simulink model "gm_uz_SVPWM_6ph"  (R2024a)
settings: Solver=FixedStepDiscrete  StartTime=0.0  StopTime=0.0004  RelTol=1e-3
undefined symbols (not defined in the file or in its folder): f_FPGA_clk, T_FPGA_clk
libraries: hdlsllib x7, simulink x1
(part 2 of 2)

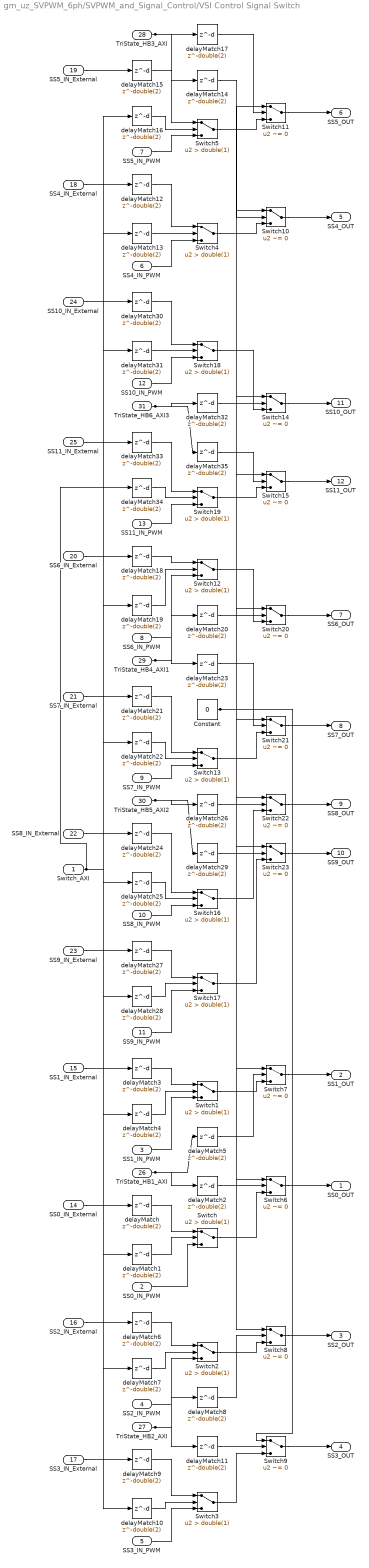
== system gm_uz_SVPWM_6ph/SVPWM_and_Signal_Control/VSI Control Signal Switch ==
  Switch_AXI : Inport  OutDataTypeStr=fixdt(0, 2, 0)  PortDimensions=1  SampleTime=1e-08
  SS0_IN_PWM : Inport  Port=2  OutDataTypeStr=fixdt(0, 1, 0)  PortDimensions=1  SampleTime=1e-08
  SS1_IN_PWM : Inport  Port=3  OutDataTypeStr=fixdt(0, 1, 0)  PortDimensions=1  SampleTime=1e-08
  SS2_IN_PWM : Inport  Port=4  OutDataTypeStr=fixdt(0, 1, 0)  PortDimensions=1  SampleTime=1e-08
  SS3_IN_PWM : Inport  Port=5  OutDataTypeStr=fixdt(0, 1, 0)  PortDimensions=1  SampleTime=1e-08
  SS4_IN_PWM : Inport  Port=6  OutDataTypeStr=fixdt(0, 1, 0)  PortDimensions=1  SampleTime=1e-08
  SS5_IN_PWM : Inport  Port=7  OutDataTypeStr=fixdt(0, 1, 0)  PortDimensions=1  SampleTime=1e-08
  SS6_IN_PWM : Inport  Port=8  OutDataTypeStr=fixdt(0, 1, 0)  PortDimensions=1  SampleTime=1e-08
  SS7_IN_PWM : Inport  Port=9  OutDataTypeStr=fixdt(0, 1, 0)  PortDimensions=1  SampleTime=1e-08
  SS8_IN_PWM : Inport  Port=10  OutDataTypeStr=fixdt(0, 1, 0)  PortDimensions=1  SampleTime=1e-08
  SS9_IN_PWM : Inport  Port=11  OutDataTypeStr=fixdt(0, 1, 0)  PortDimensions=1  SampleTime=1e-08
  SS10_IN_PWM : Inport  Port=12  OutDataTypeStr=fixdt(0, 1, 0)  PortDimensions=1  SampleTime=1e-08
  SS11_IN_PWM : Inport  Port=13  OutDataTypeStr=fixdt(0, 1, 0)  PortDimensions=1  SampleTime=1e-08
  SS0_IN_External : Inport  Port=14  OutDataTypeStr=boolean  PortDimensions=1  SampleTime=1e-08
  SS1_IN_External : Inport  Port=15  OutDataTypeStr=boolean  PortDimensions=1  SampleTime=1e-08
  SS2_IN_External : Inport  Port=16  OutDataTypeStr=boolean  PortDimensions=1  SampleTime=1e-08
  SS3_IN_External : Inport  Port=17  OutDataTypeStr=boolean  PortDimensions=1  SampleTime=1e-08
  SS4_IN_External : Inport  Port=18  OutDataTypeStr=boolean  PortDimensions=1  SampleTime=1e-08
  SS5_IN_External : Inport  Port=19  OutDataTypeStr=boolean  PortDimensions=1  SampleTime=1e-08
  SS6_IN_External : Inport  Port=20  OutDataTypeStr=boolean  PortDimensions=1  SampleTime=1e-08
  SS7_IN_External : Inport  Port=21  OutDataTypeStr=boolean  PortDimensions=1  SampleTime=1e-08
  SS8_IN_External : Inport  Port=22  OutDataTypeStr=boolean  PortDimensions=1  SampleTime=1e-08
  SS9_IN_External : Inport  Port=23  OutDataTypeStr=boolean  PortDimensions=1  SampleTime=1e-08
  SS10_IN_External : Inport  Port=24  OutDataTypeStr=boolean  PortDimensions=1  SampleTime=1e-08
  SS11_IN_External : Inport  Port=25  OutDataTypeStr=boolean  PortDimensions=1  SampleTime=1e-08
  TriState_HB1_AXI : Inport  Port=26  OutDataTypeStr=boolean  PortDimensions=1  SampleTime=1e-08
  TriState_HB2_AXI : Inport  Port=27  OutDataTypeStr=boolean  PortDimensions=1  SampleTime=1e-08
  TriState_HB3_AXI : Inport  Port=28  OutDataTypeStr=boolean  PortDimensions=1  SampleTime=1e-08
  TriState_HB4_AXI1 : Inport  Port=29  OutDataTypeStr=boolean  PortDimensions=1  SampleTime=1e-08
  TriState_HB5_AXI2 : Inport  Port=30  OutDataTypeStr=boolean  PortDimensions=1  SampleTime=1e-08
  TriState_HB6_AXI3 : Inport  Port=31  OutDataTypeStr=boolean  PortDimensions=1  SampleTime=1e-08
  Constant : Constant  Value=0  OutDataTypeStr=boolean  SampleTime=1e-08
  Switch{,1..5,12..13,16..19} (12 alike) : Switch  Criteria=u2 > Threshold  Threshold=double(1)  OutDataTypeStr=boolean  SampleTime=1e-08  SaturateOnIntegerOverflow=off  InputSameDT=off
  Switch{6..11,14..15,20..23} (12 alike) : Switch  Criteria=u2 ~= 0  Threshold=double(0)  OutDataTypeStr=boolean  SampleTime=1e-08  SaturateOnIntegerOverflow=off  InputSameDT=off
  delayMatch{,1..35} (36 alike) : Delay  DelayLength=double(2)  InitialCondition=0  SampleTime=1e-08
  SS0_OUT : Outport  SampleTime=1e-08  VectorParamsAs1DForOutWhenUnconnected=off
  SS1_OUT : Outport  Port=2  SampleTime=1e-08  VectorParamsAs1DForOutWhenUnconnected=off
  SS2_OUT : Outport  Port=3  SampleTime=1e-08  VectorParamsAs1DForOutWhenUnconnected=off
  SS3_OUT : Outport  Port=4  SampleTime=1e-08  VectorParamsAs1DForOutWhenUnconnected=off
  SS4_OUT : Outport  Port=5  SampleTime=1e-08  VectorParamsAs1DForOutWhenUnconnected=off
  SS5_OUT : Outport  Port=6  SampleTime=1e-08  VectorParamsAs1DForOutWhenUnconnected=off
  SS6_OUT : Outport  Port=7  SampleTime=1e-08  VectorParamsAs1DForOutWhenUnconnected=off
  SS7_OUT : Outport  Port=8  SampleTime=1e-08  VectorParamsAs1DForOutWhenUnconnected=off
  SS8_OUT : Outport  Port=9  SampleTime=1e-08  VectorParamsAs1DForOutWhenUnconnected=off
  SS9_OUT : Outport  Port=10  SampleTime=1e-08  VectorParamsAs1DForOutWhenUnconnected=off
  SS10_OUT : Outport  Port=11  SampleTime=1e-08  VectorParamsAs1DForOutWhenUnconnected=off
  SS11_OUT : Outport  Port=12  SampleTime=1e-08  VectorParamsAs1DForOutWhenUnconnected=off
  wires:
  delayMatch1/1 -> Switch/2
  SS0_IN_PWM/1 -> Switch/3
  SS1_IN_PWM/1 -> Switch1/3
  SS2_IN_PWM/1 -> Switch2/3
  SS3_IN_PWM/1 -> Switch3/3
  SS4_IN_PWM/1 -> Switch4/3
  SS5_IN_PWM/1 -> Switch5/3
  SS6_IN_PWM/1 -> Switch12/3
  SS7_IN_PWM/1 -> Switch13/3
  SS8_IN_PWM/1 -> Switch16/3
  SS9_IN_PWM/1 -> Switch17/3
  SS10_IN_PWM/1 -> Switch18/3
  SS11_IN_PWM/1 -> Switch19/3
  delayMatch/1 -> Switch/1
  delayMatch3/1 -> Switch1/1
  delayMatch6/1 -> Switch2/1
  delayMatch9/1 -> Switch3/1
  delayMatch12/1 -> Switch4/1
  delayMatch15/1 -> Switch5/1
  delayMatch18/1 -> Switch12/1
  delayMatch21/1 -> Switch13/1
  delayMatch24/1 -> Switch16/1
  delayMatch27/1 -> Switch17/1
  delayMatch30/1 -> Switch18/1
  delayMatch33/1 -> Switch19/1
  delayMatch2/1 -> Switch6/2
  delayMatch8/1 -> Switch8/2
  delayMatch14/1 -> Switch10/2
  delayMatch20/1 -> Switch20/2
  delayMatch26/1 -> Switch22/2
  delayMatch32/1 -> Switch14/2
  Constant/1 -> Switch9/1, Switch8/1, Switch7/1, Switch6/1, Switch23/1, Switch22/1, Switch21/1, Switch20/1, Switch15/1, Switch14/1, Switch11/1, Switch10/1
  Switch/1 -> Switch6/3
  Switch1/1 -> Switch7/3
  Switch10/1 -> SS4_OUT/1
  Switch11/1 -> SS5_OUT/1
  Switch12/1 -> Switch20/3
  Switch13/1 -> Switch21/3
  Switch14/1 -> SS10_OUT/1
  Switch15/1 -> SS11_OUT/1
  Switch16/1 -> Switch22/3
  Switch17/1 -> Switch23/3
  Switch18/1 -> Switch14/3
  Switch19/1 -> Switch15/3
  Switch2/1 -> Switch8/3
  Switch20/1 -> SS6_OUT/1
  Switch21/1 -> SS7_OUT/1
  Switch22/1 -> SS8_OUT/1
  Switch23/1 -> SS9_OUT/1
  Switch3/1 -> Switch9/3
  Switch4/1 -> Switch10/3
  Switch5/1 -> Switch11/3
  Switch6/1 -> SS0_OUT/1
  Switch7/1 -> SS1_OUT/1
  Switch8/1 -> SS2_OUT/1
  Switch9/1 -> SS3_OUT/1
  SS0_IN_External/1 -> delayMatch/1
  delayMatch4/1 -> Switch1/2
  delayMatch5/1 -> Switch7/2
  SS1_IN_External/1 -> delayMatch3/1
  delayMatch7/1 -> Switch2/2
  TriState_HB1_AXI/1 -> delayMatch5/1, delayMatch2/1
  SS2_IN_External/1 -> delayMatch6/1
  delayMatch10/1 -> Switch3/2
  delayMatch11/1 -> Switch9/2
  SS3_IN_External/1 -> delayMatch9/1
  delayMatch13/1 -> Switch4/2
  TriState_HB2_AXI/1 -> delayMatch11/1, delayMatch8/1
  SS4_IN_External/1 -> delayMatch12/1
  delayMatch16/1 -> Switch5/2
  delayMatch17/1 -> Switch11/2
  SS5_IN_External/1 -> delayMatch15/1
  delayMatch19/1 -> Switch12/2
  TriState_HB3_AXI/1 -> delayMatch17/1, delayMatch14/1
  SS6_IN_External/1 -> delayMatch18/1
  delayMatch22/1 -> Switch13/2
  delayMatch23/1 -> Switch21/2
  SS7_IN_External/1 -> delayMatch21/1
  delayMatch25/1 -> Switch16/2
  TriState_HB4_AXI1/1 -> delayMatch23/1, delayMatch20/1
  SS8_IN_External/1 -> delayMatch24/1
  delayMatch28/1 -> Switch17/2
  delayMatch29/1 -> Switch23/2
  SS9_IN_External/1 -> delayMatch27/1
  delayMatch31/1 -> Switch18/2
  TriState_HB5_AXI2/1 -> delayMatch29/1, delayMatch26/1
  SS10_IN_External/1 -> delayMatch30/1
  delayMatch34/1 -> Switch19/2
  delayMatch35/1 -> Switch15/2
  SS11_IN_External/1 -> delayMatch33/1
  Switch_AXI/1 -> delayMatch34/1, delayMatch31/1, delayMatch28/1, delayMatch25/1, delayMatch22/1, delayMatch19/1, delayMatch16/1, delayMatch13/1, delayMatch10/1, delayMatch7/1, delayMatch4/1, delayMatch1/1
  TriState_HB6_AXI3/1 -> delayMatch35/1, delayMatch32/1

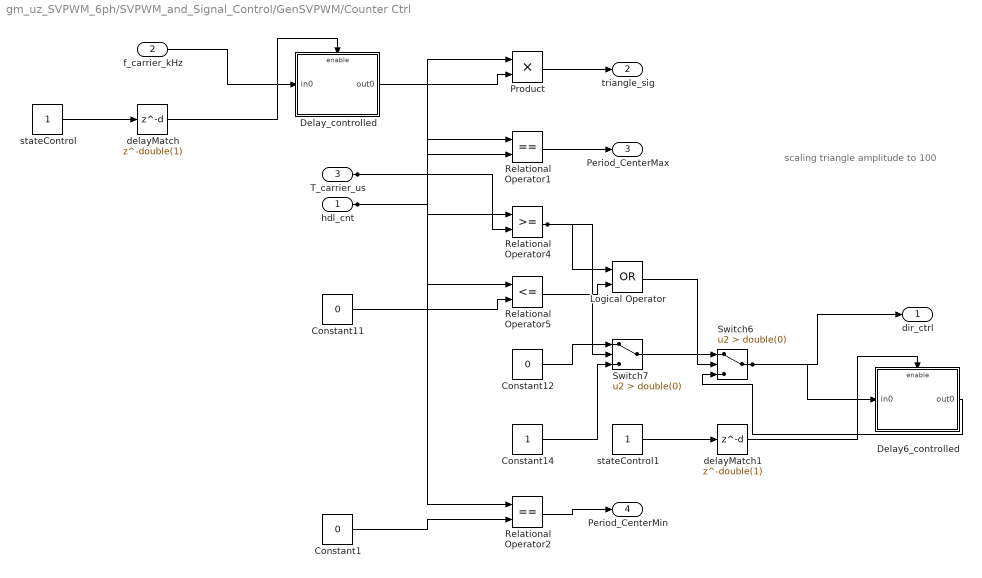
== system gm_uz_SVPWM_6ph/SVPWM_and_Signal_Control/GenSVPWM/Counter Ctrl ==
  note: scaling triangle amplitude to 100
  hdl_cnt : Inport  OutDataTypeStr=fixdt(0, 20, 0)  PortDimensions=1  SampleTime=1e-08
  f_carrier_kHz : Inport  Port=2  OutDataTypeStr=fixdt(0, 25, 26)  PortDimensions=1  SampleTime=1e-08
  T_carrier_us : Inport  Port=3  OutDataTypeStr=fixdt(0, 25, 0)  PortDimensions=1  SampleTime=1e-08
  Constant1 : Constant  Value=0  OutDataTypeStr=fixdt(0, 20, 0)  SampleTime=1e-08
  Constant11 : Constant  Value=0  OutDataTypeStr=fixdt(0, 20, 0)  SampleTime=1e-08
  Constant12 : Constant  Value=0  OutDataTypeStr=boolean  SampleTime=1e-08
  Constant14 : Constant  OutDataTypeStr=boolean  SampleTime=1e-08
  Delay6_controlled : Subsystem
  Delay_controlled : Subsystem
  Logical Operator : Logic  Operator=OR  AllPortsSameDT=off  OutDataTypeStr=boolean  SampleTime=1e-08
  Product : Product  Inputs=**  OutDataTypeStr=fixdt(0, 18, 17)  SampleTime=1e-08
  Relational Operator1 : RelationalOperator  Operator===  OutDataTypeStr=boolean  SampleTime=1e-08  InputSameDT=off
  Relational Operator2 : RelationalOperator  Operator===  OutDataTypeStr=boolean  SampleTime=1e-08  InputSameDT=off
  Relational Operator4 : RelationalOperator  OutDataTypeStr=boolean  SampleTime=1e-08  InputSameDT=off
  Relational Operator5 : RelationalOperator  Operator=<=  OutDataTypeStr=boolean  SampleTime=1e-08  InputSameDT=off
  Switch6 : Switch  Criteria=u2 > Threshold  Threshold=double(0)  OutDataTypeStr=boolean  SampleTime=1e-08  SaturateOnIntegerOverflow=off  InputSameDT=off
  Switch7 : Switch  Criteria=u2 > Threshold  Threshold=double(0)  OutDataTypeStr=boolean  SampleTime=1e-08  SaturateOnIntegerOverflow=off  InputSameDT=off
  delayMatch : Delay  DelayLength=double(1)  InitialCondition=0  SampleTime=1e-08
  delayMatch1 : Delay  DelayLength=double(1)  InitialCondition=0  SampleTime=1e-08
  stateControl : Constant  OutDataTypeStr=boolean  SampleTime=1e-08
  stateControl1 : Constant  OutDataTypeStr=boolean  SampleTime=1e-08
  dir_ctrl : Outport  SampleTime=1e-08  VectorParamsAs1DForOutWhenUnconnected=off
  triangle_sig : Outport  Port=2  SampleTime=1e-08  VectorParamsAs1DForOutWhenUnconnected=off
  Period_CenterMax : Outport  Port=3  SampleTime=1e-08  VectorParamsAs1DForOutWhenUnconnected=off
  Period_CenterMin : Outport  Port=4  SampleTime=1e-08  VectorParamsAs1DForOutWhenUnconnected=off
  wires:
  hdl_cnt/1 -> Relational Operator5/1, Relational Operator4/1, Relational Operator2/1, Relational Operator1/1, Product/1
  f_carrier_kHz/1 -> Delay_controlled/1(in0)
  T_carrier_us/1 -> Relational Operator4/2, Relational Operator1/2
  Constant1/1 -> Relational Operator2/2
  Constant11/1 -> Relational Operator5/2
  Constant12/1 -> Switch7/1
  Constant14/1 -> Switch7/3
  Delay_controlled/1(out0) -> Product/2
  Product/1 -> triangle_sig/1
  Relational Operator1/1 -> Period_CenterMax/1
  Relational Operator2/1 -> Period_CenterMin/1
  Relational Operator4/1 -> Switch7/2, Logical Operator/1
  Relational Operator5/1 -> Logical Operator/2
  Switch6/1 -> dir_ctrl/1, Delay6_controlled/1(in0)
  delayMatch/1 -> Delay_controlled/Enable
  Delay6_controlled/1(out0) -> Switch6/3
  delayMatch1/1 -> Delay6_controlled/Enable
  Switch7/1 -> Switch6/1
  Logical Operator/1 -> Switch6/2
  stateControl/1 -> delayMatch/1
  stateControl1/1 -> delayMatch1/1

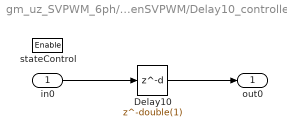
== system gm_uz_SVPWM_6ph/SVPWM_and_Signal_Control/GenSVPWM/Delay10_controlled ==
  in0 : Inport  OutDataTypeStr=fixdt(0, 6, 0)  SampleTime=1e-08
  stateControl : EnablePort  OutDataTypeStr=boolean
  Delay10 : Delay  DelayLength=double(1)  InitialCondition=0  SampleTime=1e-08
  out0 : Outport  OutDataTypeStr=fixdt(0, 6, 0)  SampleTime=1e-08
  wires:
  Delay10/1 -> out0/1
  in0/1 -> Delay10/1

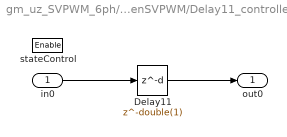
== system gm_uz_SVPWM_6ph/SVPWM_and_Signal_Control/GenSVPWM/Delay11_controlled ==
  in0 : Inport  OutDataTypeStr=fixdt(0, 6, 0)  SampleTime=1e-08
  stateControl : EnablePort  OutDataTypeStr=boolean
  Delay11 : Delay  DelayLength=double(1)  InitialCondition=0  SampleTime=1e-08
  out0 : Outport  OutDataTypeStr=fixdt(0, 6, 0)  SampleTime=1e-08
  wires:
  Delay11/1 -> out0/1
  in0/1 -> Delay11/1

== system gm_uz_SVPWM_6ph/SVPWM_and_Signal_Control/GenSVPWM/Delay12_controlled ==
  in0 : Inport  OutDataTypeStr=fixdt(0, 6, 0)  SampleTime=1e-08
  stateControl : EnablePort  OutDataTypeStr=boolean
  Delay12 : Delay  DelayLength=double(1)  InitialCondition=0  SampleTime=1e-08
  out0 : Outport  OutDataTypeStr=fixdt(0, 6, 0)  SampleTime=1e-08
  wires:
  Delay12/1 -> out0/1
  in0/1 -> Delay12/1

== system gm_uz_SVPWM_6ph/SVPWM_and_Signal_Control/GenSVPWM/Delay1_controlled ==
  in0 : Inport  OutDataTypeStr=fixdt(1, 18, 16)  SampleTime=1e-08
  stateControl : EnablePort  OutDataTypeStr=boolean
  Delay1 : Delay  DelayLength=double(1)  InitialCondition=0  SampleTime=1e-08
  out0 : Outport  OutDataTypeStr=fixdt(1, 18, 16)  SampleTime=1e-08
  wires:
  Delay1/1 -> out0/1
  in0/1 -> Delay1/1

== system gm_uz_SVPWM_6ph/SVPWM_and_Signal_Control/GenSVPWM/Delay2_controlled ==
  in0 : Inport  OutDataTypeStr=fixdt(1, 18, 16)  SampleTime=1e-08
  stateControl : EnablePort  OutDataTypeStr=boolean
  Delay2 : Delay  DelayLength=double(1)  InitialCondition=0  SampleTime=1e-08
  out0 : Outport  OutDataTypeStr=fixdt(1, 18, 16)  SampleTime=1e-08
  wires:
  Delay2/1 -> out0/1
  in0/1 -> Delay2/1

== system gm_uz_SVPWM_6ph/SVPWM_and_Signal_Control/GenSVPWM/Delay5_controlled ==
  in0 : Inport  OutDataTypeStr=fixdt(1, 18, 16)  SampleTime=1e-08
  stateControl : EnablePort  OutDataTypeStr=boolean
  Delay5 : Delay  DelayLength=double(1)  InitialCondition=0  SampleTime=1e-08
  out0 : Outport  OutDataTypeStr=fixdt(1, 18, 16)  SampleTime=1e-08
  wires:
  Delay5/1 -> out0/1
  in0/1 -> Delay5/1

== system gm_uz_SVPWM_6ph/SVPWM_and_Signal_Control/GenSVPWM/Delay6_controlled ==
  in0 : Inport  OutDataTypeStr=fixdt(1, 18, 16)  SampleTime=1e-08
  stateControl : EnablePort  OutDataTypeStr=boolean
  Delay6 : Delay  DelayLength=double(1)  InitialCondition=0  SampleTime=1e-08
  out0 : Outport  OutDataTypeStr=fixdt(1, 18, 16)  SampleTime=1e-08
  wires:
  Delay6/1 -> out0/1
  in0/1 -> Delay6/1

== system gm_uz_SVPWM_6ph/SVPWM_and_Signal_Control/GenSVPWM/Delay8_controlled ==
  in0 : Inport  OutDataTypeStr=fixdt(0, 6, 0)  SampleTime=1e-08
  stateControl : EnablePort  OutDataTypeStr=boolean
  Delay8 : Delay  DelayLength=double(1)  InitialCondition=0  SampleTime=1e-08
  out0 : Outport  OutDataTypeStr=fixdt(0, 6, 0)  SampleTime=1e-08
  wires:
  Delay8/1 -> out0/1
  in0/1 -> Delay8/1

== system gm_uz_SVPWM_6ph/SVPWM_and_Signal_Control/GenSVPWM/Delay9_controlled ==
  in0 : Inport  OutDataTypeStr=fixdt(0, 6, 0)  SampleTime=1e-08
  stateControl : EnablePort  OutDataTypeStr=boolean
  Delay9 : Delay  DelayLength=double(1)  InitialCondition=0  SampleTime=1e-08
  out0 : Outport  OutDataTypeStr=fixdt(0, 6, 0)  SampleTime=1e-08
  wires:
  Delay9/1 -> out0/1
  in0/1 -> Delay9/1

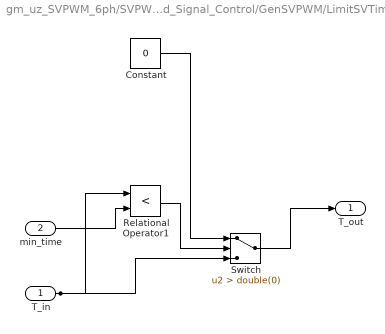
== system gm_uz_SVPWM_6ph/SVPWM_and_Signal_Control/GenSVPWM/LimitSVTime ==
  T_in : Inport  OutDataTypeStr=fixdt(1, 18, 16)  PortDimensions=1  SampleTime=1e-08
  min_time : Inport  Port=2  OutDataTypeStr=fixdt(1, 18, 16)  PortDimensions=1  SampleTime=1e-08
  Constant : Constant  Value=0  OutDataTypeStr=fixdt(1, 18, 16)  SampleTime=1e-08
  Relational Operator1 : RelationalOperator  Operator=<  OutDataTypeStr=boolean  SampleTime=1e-08  InputSameDT=off
  Switch : Switch  Criteria=u2 > Threshold  Threshold=double(0)  OutDataTypeStr=fixdt(1, 18, 16)  SampleTime=1e-08  SaturateOnIntegerOverflow=off  InputSameDT=off
  T_out : Outport  SampleTime=1e-08  VectorParamsAs1DForOutWhenUnconnected=off
  wires:
  T_in/1 -> Switch/3, Relational Operator1/1
  min_time/1 -> Relational Operator1/2
  Constant/1 -> Switch/1
  Relational Operator1/1 -> Switch/2
  Switch/1 -> T_out/1

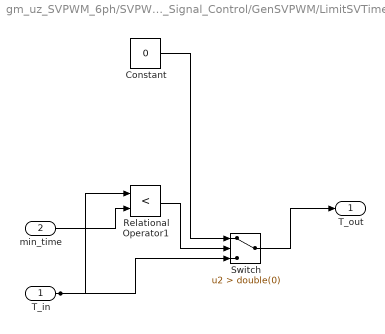
== system gm_uz_SVPWM_6ph/SVPWM_and_Signal_Control/GenSVPWM/LimitSVTime1 ==
  T_in : Inport  OutDataTypeStr=fixdt(1, 18, 16)  PortDimensions=1  SampleTime=1e-08
  min_time : Inport  Port=2  OutDataTypeStr=fixdt(1, 18, 16)  PortDimensions=1  SampleTime=1e-08
  Constant : Constant  Value=0  OutDataTypeStr=fixdt(1, 18, 16)  SampleTime=1e-08
  Relational Operator1 : RelationalOperator  Operator=<  OutDataTypeStr=boolean  SampleTime=1e-08  InputSameDT=off
  Switch : Switch  Criteria=u2 > Threshold  Threshold=double(0)  OutDataTypeStr=fixdt(1, 18, 16)  SampleTime=1e-08  SaturateOnIntegerOverflow=off  InputSameDT=off
  T_out : Outport  SampleTime=1e-08  VectorParamsAs1DForOutWhenUnconnected=off
  wires:
  T_in/1 -> Switch/3, Relational Operator1/1
  min_time/1 -> Relational Operator1/2
  Constant/1 -> Switch/1
  Relational Operator1/1 -> Switch/2
  Switch/1 -> T_out/1

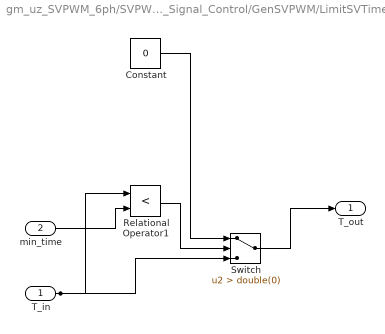
== system gm_uz_SVPWM_6ph/SVPWM_and_Signal_Control/GenSVPWM/LimitSVTime2 ==
  T_in : Inport  OutDataTypeStr=fixdt(1, 18, 16)  PortDimensions=1  SampleTime=1e-08
  min_time : Inport  Port=2  OutDataTypeStr=fixdt(1, 18, 16)  PortDimensions=1  SampleTime=1e-08
  Constant : Constant  Value=0  OutDataTypeStr=fixdt(1, 18, 16)  SampleTime=1e-08
  Relational Operator1 : RelationalOperator  Operator=<  OutDataTypeStr=boolean  SampleTime=1e-08  InputSameDT=off
  Switch : Switch  Criteria=u2 > Threshold  Threshold=double(0)  OutDataTypeStr=fixdt(1, 18, 16)  SampleTime=1e-08  SaturateOnIntegerOverflow=off  InputSameDT=off
  T_out : Outport  SampleTime=1e-08  VectorParamsAs1DForOutWhenUnconnected=off
  wires:
  T_in/1 -> Switch/3, Relational Operator1/1
  min_time/1 -> Relational Operator1/2
  Constant/1 -> Switch/1
  Relational Operator1/1 -> Switch/2
  Switch/1 -> T_out/1

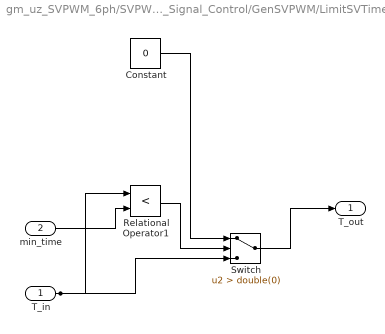
== system gm_uz_SVPWM_6ph/SVPWM_and_Signal_Control/GenSVPWM/LimitSVTime3 ==
  T_in : Inport  OutDataTypeStr=fixdt(1, 18, 16)  PortDimensions=1  SampleTime=1e-08
  min_time : Inport  Port=2  OutDataTypeStr=fixdt(1, 18, 16)  PortDimensions=1  SampleTime=1e-08
  Constant : Constant  Value=0  OutDataTypeStr=fixdt(1, 18, 16)  SampleTime=1e-08
  Relational Operator1 : RelationalOperator  Operator=<  OutDataTypeStr=boolean  SampleTime=1e-08  InputSameDT=off
  Switch : Switch  Criteria=u2 > Threshold  Threshold=double(0)  OutDataTypeStr=fixdt(1, 18, 16)  SampleTime=1e-08  SaturateOnIntegerOverflow=off  InputSameDT=off
  T_out : Outport  SampleTime=1e-08  VectorParamsAs1DForOutWhenUnconnected=off
  wires:
  T_in/1 -> Switch/3, Relational Operator1/1
  min_time/1 -> Relational Operator1/2
  Constant/1 -> Switch/1
  Relational Operator1/1 -> Switch/2
  Switch/1 -> T_out/1

== system gm_uz_SVPWM_6ph/SVPWM_and_Signal_Control/GenSVPWM/Counter Ctrl/Delay6_controlled ==
  in0 : Inport  OutDataTypeStr=boolean  SampleTime=1e-08
  stateControl : EnablePort  OutDataTypeStr=boolean
  Delay6 : Delay  DelayLength=double(1)  InitialCondition=0  SampleTime=1e-08
  out0 : Outport  OutDataTypeStr=boolean  SampleTime=1e-08
  wires:
  Delay6/1 -> out0/1
  in0/1 -> Delay6/1

== system gm_uz_SVPWM_6ph/SVPWM_and_Signal_Control/GenSVPWM/Counter Ctrl/Delay_controlled ==
  in0 : Inport  OutDataTypeStr=fixdt(0, 25, 26)  SampleTime=1e-08
  stateControl : EnablePort  OutDataTypeStr=boolean
  Delay : Delay  DelayLength=double(1)  InitialCondition=0  SampleTime=1e-08
  out0 : Outport  OutDataTypeStr=fixdt(0, 25, 26)  SampleTime=1e-08
  wires:
  Delay/1 -> out0/1
  in0/1 -> Delay/1
